simulink model "Quad_IGE_Landing_PF"  (R2023b)
settings: Solver=ode4  StartTime=0.0  StopTime=20  FixedStep=0.01  RelTol=1e-3
InitFcn:
  | m = 0.063;
  | g = 9.81;
  | R = 0.033;
  | h_r = 0.013;
  | b = 0.2;
libraries: simulink x2
settings Model: Creator=reza  LastModifiedBy=Ali
settings OptimizationCC: ReuseModelBlockBuffer=off

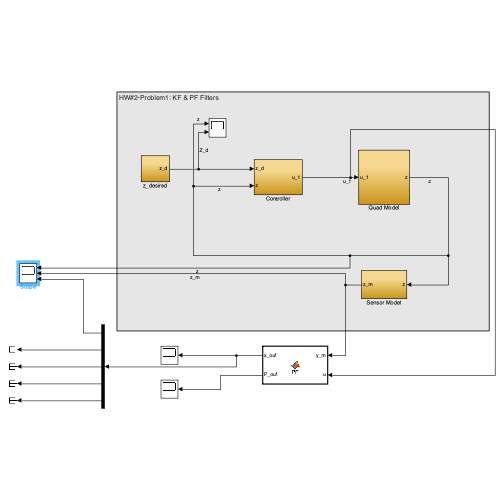
[thumbnail: Simulink's stored preview of the top-level diagram]
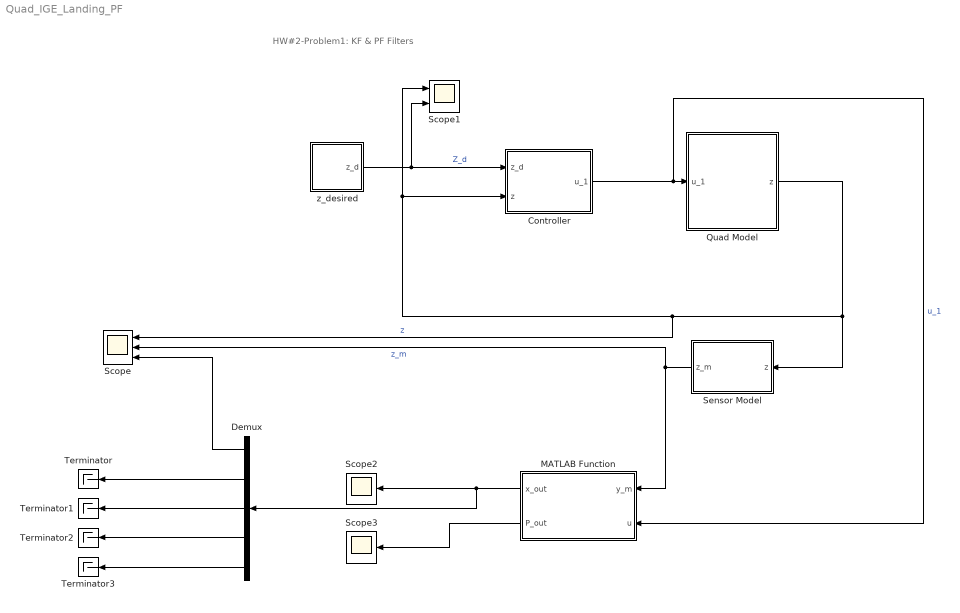
== system Quad_IGE_Landing_PF ==
  note: HW#2-Problem1: KF & PF Filters
  Controller : Subsystem
  Demux : Demux  Outputs=5
  MATLAB Function : MATLAB Function  TreatAsAtomicUnit=on
  Quad Model : Subsystem
  Scope : Scope  NumInputPorts=3
  Scope1 : Scope  NumInputPorts=2
  Scope2 : Scope
  Scope3 : Scope
  Sensor Model : Subsystem
  Terminator{,1..3} (4 alike) : Terminator
  z_desired : Subsystem
  wires:
  Quad Model/1(z) -> Scope/1, Scope1/1, Controller/2(z), Sensor Model/1(z)  "z"
  z_desired/1(z_d) -> Scope1/2, Controller/1(z_d)  "Z_d"
  Sensor Model/1(z_m) -> MATLAB Function/1(y_m), Scope/2  "z_m"
  Controller/1(u_1) -> MATLAB Function/2(u), Quad Model/1(u_1)  "u_1"
  MATLAB Function/1(x_out) -> Demux/1, Scope2/1
  MATLAB Function/2(P_out) -> Scope3/1
  Demux/1 -> Scope/3
  Demux/2 -> Terminator/1
  Demux/3 -> Terminator1/1
  Demux/4 -> Terminator2/1
  Demux/5 -> Terminator3/1

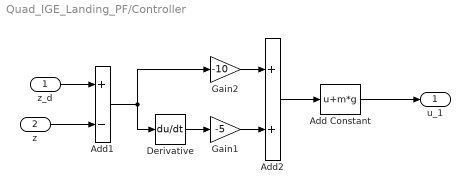
== system Quad_IGE_Landing_PF/Controller ==
  z_d : Inport
  z : Inport  Port=2
  Add Constant : Bias  Bias=m*g  SaturateOnIntegerOverflow=off
  Add1 : Sum  Inputs=+-
  Add2 : Sum
  Derivative : Derivative
  Gain1 : Gain  Gain=-5
  Gain2 : Gain  Gain=-10
  u_1 : Outport
  wires:
  Gain1/1 -> Add2/2
  Add2/1 -> Add Constant/1
  z_d/1 -> Add1/1
  Add1/1 -> Gain2/1, Derivative/1
  Gain2/1 -> Add2/1
  Derivative/1 -> Gain1/1
  Add Constant/1 -> u_1/1
  z/1 -> Add1/2

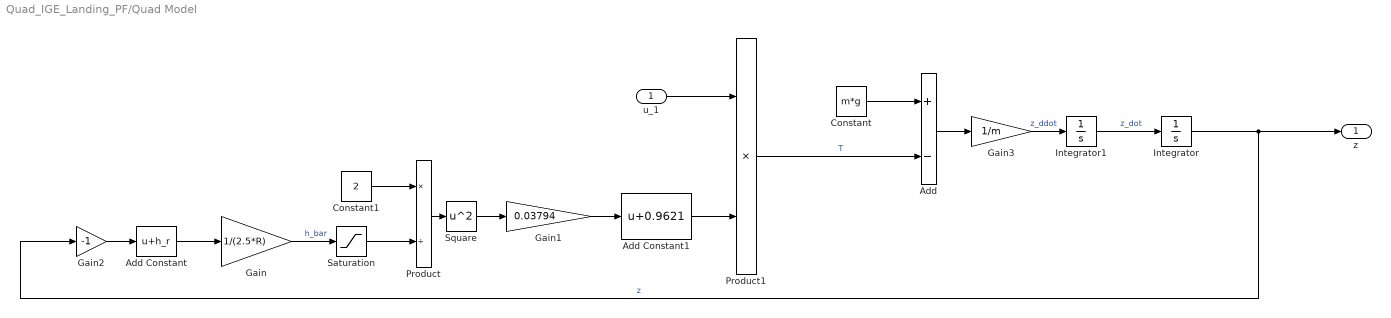
== system Quad_IGE_Landing_PF/Quad Model ==
  u_1 : Inport
  Add : Sum  Inputs=+-
  Add Constant : Bias  Bias=h_r  SaturateOnIntegerOverflow=off
  Add Constant1 : Bias  Bias=0.9621  SaturateOnIntegerOverflow=off
  Constant : Constant  Value=m*g
  Constant1 : Constant  Value=2
  Gain : Gain  Gain=1/(2.5*R)
  Gain1 : Gain  Gain=0.03794
  Gain2 : Gain  Gain=-1
  Gain3 : Gain  Gain=1/m
  Integrator : Integrator  InitialCondition=-2
  Integrator1 : Integrator
  Product : Product  Inputs=*/
  Product1 : Product
  Saturation : Saturate  UpperLimit=2  LowerLimit=0
  Square : Math  Operator=square
  z : Outport
  wires:
  Saturation/1 -> Product/2
  Integrator1/1 -> Integrator/1  "z_dot"
  Gain/1 -> Saturation/1  "h_bar"
  Add/1 -> Gain3/1
  Add Constant/1 -> Gain/1
  Integrator/1 -> Gain2/1, z/1  "z"
  Gain1/1 -> Add Constant1/1
  Product/1 -> Square/1
  Square/1 -> Gain1/1
  Add Constant1/1 -> Product1/2
  Constant/1 -> Add/1
  Constant1/1 -> Product/1
  Product1/1 -> Add/2  "T"
  u_1/1 -> Product1/1
  Gain2/1 -> Add Constant/1
  Gain3/1 -> Integrator1/1  "z_ddot"

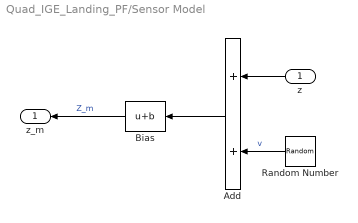
== system Quad_IGE_Landing_PF/Sensor Model ==
  z : Inport
  Add : Sum
  Bias : Bias  Bias=b  SaturateOnIntegerOverflow=off
  Random Number : RandomNumber  Variance=0.1  SampleTime=0.01
  z_m : Outport
  wires:
  Random Number/1 -> Add/2  "v"
  Add/1 -> Bias/1
  z/1 -> Add/1
  Bias/1 -> z_m/1  "Z_m"

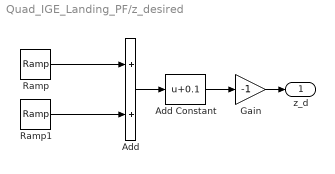
== system Quad_IGE_Landing_PF/z_desired ==
  Add : Sum
  Add Constant : Bias  Bias=0.1  SaturateOnIntegerOverflow=off
  Gain : Gain  Gain=-1
  Ramp : simulink/Sources/Ramp  slope=-(2-0.1)/5  start=10  InitialOutput=2-0.1
  Ramp1 : simulink/Sources/Ramp  slope=(2-0.1)/5  start=15  InitialOutput=0
  z_d : Outport
  wires:
  Add Constant/1 -> Gain/1
  Ramp1/1 -> Add/2
  Ramp/1 -> Add/1
  Add/1 -> Add Constant/1
  Gain/1 -> z_d/1

== matlab function Quad_IGE_Landing_PF/MATLAB Function ==
  settings: updateMethod=DISCRETE
  data: y_m input; x_out output; u input; P_out output
function [x_out,P_out] = PF(y_m,u)

%constant parameters
m = 0.063;
g = 9.81;
r = 0.033;
h_r = 0.013;
b = 0.2;
Ts = 0.01;

Q = diag([0.1,1,10e-20,10e-20,10e-20]);
R = 10e-2;
N=100;
persistent P
if isempty(P)
    P = diag([1,1,0.1,0.1,0.1]);
end
 

persistent x_hat xpart

if isempty(x_hat)
    x_hat = [-2 ;0 ;0.9621 ;0.03794 ; 0.2]; 
end

if isempty(xpart)
    xpart = zeros(5,N); 
    P_d = [P(1,1);P(2,2);P(3,3);P(4,4);P(5,5)];
    for i = 1 : N
        xpart(:,i) = x_hat + sqrt(P_d) * randn;
    end
end



%% Particle filter
q = zeros(N,1)
xpartminus = zeros(5,N);
for i = 1 : N
    xpartminus(1,i) = xpart(1,i) + Ts*xpart(2,i)+ sqrt(Q(1,1)) * randn;
    xpartminus(2,i) = xpart(2,i) + Ts*(g - 1/m*(xpart(3,i) + xpart(4,i)*(5*r/(h_r - xpart(1,i)))^2)*u)+ sqrt(Q(2,2)) * randn;
    xpartminus(3,i) = xpart(3,i)+ sqrt(Q(3,3)) * randn;
    xpartminus(4,i) = xpart(4,i)+ sqrt(Q(4,4)) * randn;
    xpartminus(5,i) = xpart(5,i)+ sqrt(Q(5,5)) * randn;

    ypart = xpartminus(1,i) + xpartminus(5,i);
    vhat = y_m - ypart;
    q(i) = (1 / sqrt(R) / sqrt(2*pi)) * exp(-vhat^2 / 2 / R);

end

%% Normalize the likelihood of each a priori estimate.
    qsum = sum(q);
    for i = 1 : N
        q(i) = q(i) / qsum;
    end

 %% Resample.
    for i = 1 : N
        u = rand; % uniform random number between 0 and 1
        qtempsum = 0;
        for j = 1 : N
            qtempsum = qtempsum + q(j);
            if qtempsum >= u
                xpart(:,i) = xpartminus(:,j);
                break;
            end
        end
    end

%% The particle filter estimate is the mean of the particles.
x_hat = mean(xpart,2);
x_out = x_hat
P_out = [P(1,1);P(2,2);P(3,3);P(4,4);P(5,5)]
